simulink library "CTRL_SPECCTRL_FF_ACCPED"  (R2024b)
settings: Solver=VariableStepAuto  StartTime=0.0  StopTime=10.0  RelTol=1e-3
undefined symbols (not defined in the file or in its folder): CTRL_SPECCTRL_FF_ACCPED_p_DmpLim_p100, CTRL_SPECCTRL_FF_ACCPED_p_DmpLoLim_p100, CTRL_SPECCTRL_FF_ACCPED_p_DmpUpLim_p100, CTRL_SPECCTRL_FF_ACCPED_p_DwlTime_s, CTRL_SPECCTRL_FF_ACCPED_p_RegBaseCoef_na, CTRL_SPECCTRL_FF_ACCPED_p_RegComCoef_na, CTRL_SPECCTRL_FF_ACCPED_p_RegSpCoef_na, CTRL_SPECCTRL_FF_ACCPED_px_PosRatThr_p100ps, CTRL_SPECCTRL_FF_ACCPED_pxy_Dmp_p100, CTRL_SPECCTRL_FF_ACCPED_py_RefSped_mps
libraries: simulink x1
settings Model: Creator=blatak  LastModifiedBy=blatak

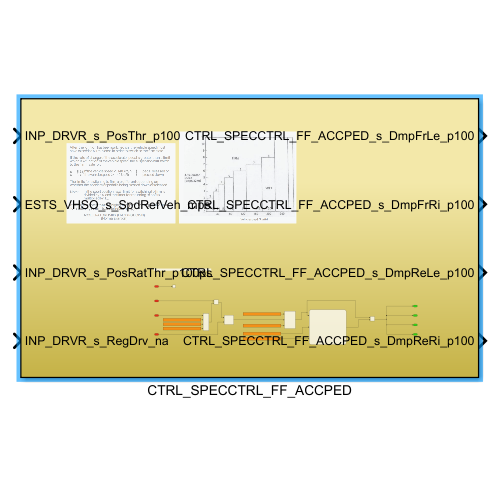
[thumbnail: Simulink's stored preview of the top-level diagram]
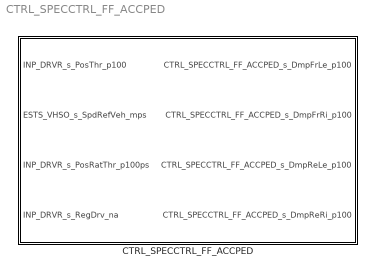
== system CTRL_SPECCTRL_FF_ACCPED ==
  CTRL_SPECCTRL_FF_ACCPED : Subsystem

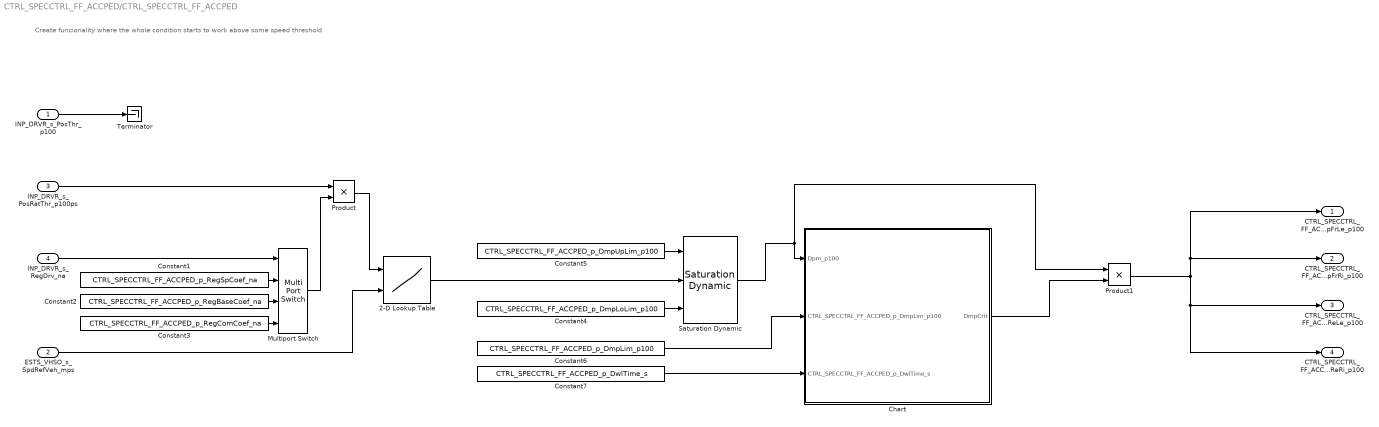
== system CTRL_SPECCTRL_FF_ACCPED/CTRL_SPECCTRL_FF_ACCPED ==
  note: Create funcionality where the whole condition starts to work above some speed threshold
  INP_DRVR_s_PosThr_p100 : Inport
  ESTS_VHSO_s_SpdRefVeh_mps : Inport  Port=2
  INP_DRVR_s_PosRatThr_p100ps : Inport  Port=3
  INP_DRVR_s_RegDrv_na : Inport  Port=4
  2-D Lookup Table : Lookup_n-D  BreakpointsForDimension1=CTRL_SPECCTRL_FF_ACCPED_px_PosRatThr_p100ps  BreakpointsForDimension2=CTRL_SPECCTRL_FF_ACCPED_py_RefSped_mps  Table=CTRL_SPECCTRL_FF_ACCPED_pxy_Dmp_p100  InternalRulePriority=Speed  RndMeth=Simplest
      settings: InputPortMap=u0,u1
  Chart : Stateflow chart  TreatAsAtomicUnit=on
  Constant1 : Constant  Value=CTRL_SPECCTRL_FF_ACCPED_p_RegSpCoef_na
  Constant2 : Constant  Value=CTRL_SPECCTRL_FF_ACCPED_p_RegBaseCoef_na
  Constant3 : Constant  Value=CTRL_SPECCTRL_FF_ACCPED_p_RegComCoef_na
  Constant4 : Constant  Value=CTRL_SPECCTRL_FF_ACCPED_p_DmpLoLim_p100
  Constant5 : Constant  Value=CTRL_SPECCTRL_FF_ACCPED_p_DmpUpLim_p100
  Constant6 : Constant  Value=CTRL_SPECCTRL_FF_ACCPED_p_DmpLim_p100
  Constant7 : Constant  Value=CTRL_SPECCTRL_FF_ACCPED_p_DwlTime_s
  Multiport Switch : MultiPortSwitch  SaturateOnIntegerOverflow=off  InputSameDT=off
  Product : Product
  Product1 : Product
  Saturation Dynamic : simulink/Discontinuities/Saturation Dynamic  OutMin=[]  OutMax=[]  OutDataTypeStr=Inherit: Same as second input  OutDataType=fixdt(1, 16)  OutScaling=2^-10  DoSatur=off
  Terminator : Terminator
  CTRL_SPECCTRL_FF_ACCPED_s_DmpFrLe_p100 : Outport
  CTRL_SPECCTRL_FF_ACCPED_s_DmpFrRi_p100 : Outport  Port=2
  CTRL_SPECCTRL_FF_ACCPED_s_DmpReLe_p100 : Outport  Port=3
  CTRL_SPECCTRL_FF_ACCPED_s_DmpReRi_p100 : Outport  Port=4
  wires:
  Product1/1 -> CTRL_SPECCTRL_FF_ACCPED_s_DmpFrRi_p100/1, CTRL_SPECCTRL_FF_ACCPED_s_DmpFrLe_p100/1, CTRL_SPECCTRL_FF_ACCPED_s_DmpReRi_p100/1, CTRL_SPECCTRL_FF_ACCPED_s_DmpReLe_p100/1
  INP_DRVR_s_PosRatThr_p100ps/1 -> Product/1
  Chart/1(DmpCrit) -> Product1/2
  Constant4/1 -> Saturation Dynamic/3
  Constant5/1 -> Saturation Dynamic/1
  Product/1 -> 2-D Lookup Table/1
  ESTS_VHSO_s_SpdRefVeh_mps/1 -> 2-D Lookup Table/2
  Saturation Dynamic/1 -> Product1/1, Chart/1(Dpm_p100)
  Multiport Switch/1 -> Product/2
  2-D Lookup Table/1 -> Saturation Dynamic/2
  INP_DRVR_s_RegDrv_na/1 -> Multiport Switch/1
  Constant1/1 -> Multiport Switch/2
  Constant2/1 -> Multiport Switch/3
  Constant3/1 -> Multiport Switch/4
  INP_DRVR_s_PosThr_p100/1 -> Terminator/1
  Constant7/1 -> Chart/3(CTRL_SPECCTRL_FF_ACCPED_p_DwlTime_s)
  Constant6/1 -> Chart/2(CTRL_SPECCTRL_FF_ACCPED_p_DmpLim_p100)

== stateflow chart CTRL_SPECCTRL_FF_ACCPED/Chart ==
  state Default
    en:DmpCrit=0;
  state Firm
    en:DmpCrit=1;
  state Base
    en:DmpCrit=0;
  (default) -> Default
  Default -> Base [order 1] : [Dpm_p100<=CTRL_SPECCTRL_FF_ACCPED_p_DmpLim_p100]
  Default -> Firm [order 2] : [Dpm_p100>CTRL_SPECCTRL_FF_ACCPED_p_DmpLim_p100]
  Firm -> Base : [duration(Dpm_p100<CTRL_SPECCTRL_FF_ACCPED_p_DmpLim_p100)>CTRL_SPECCTRL_FF_ACCPED_p_DwlTime_s]
  Base -> Firm : [Dpm_p100>CTRL_SPECCTRL_FF_ACCPED_p_DmpLim_p100]
  data: Dpm_p100 input; DmpCrit output; CTRL_SPECCTRL_FF_ACCPED_p_DmpLim_p100 input; CTRL_SPECCTRL_FF_ACCPED_p_DwlTime_s input
